simulink model "mecanique"  (Simulink 6.0)
settings: Solver=ode45  StartTime=0.0  StopTime=10.0  RelTol=1e-3
libraries: mblibv1 x11, simulink x4
settings Model: LastModifiedBy=sebastien

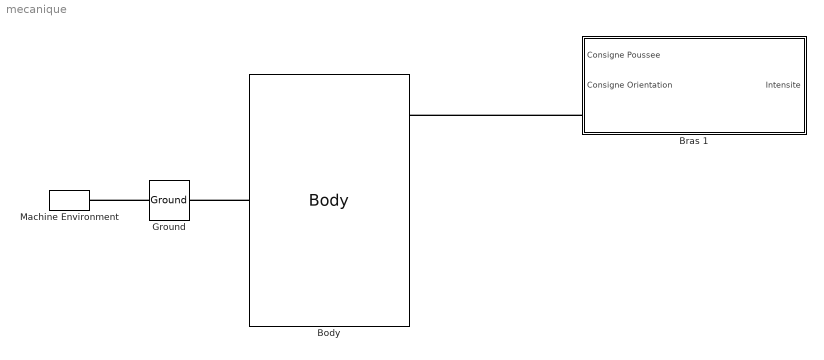
== system mecanique ==
  Body : mblibv1/Bodies/Body  PhysicalDomain=mechanical  SubClassName=Unknown  LeftPortType=workingframe  RightPortType=workingframe  LConnTagsString=CS1  RConnTagsString=CS2|CS3|CS4  DialogClass=MechanicalBodyBlock  Mass=1  MassUnits=kg  InertiaUnits=kg*m^2  Inertia=eye(3)  Shape=Cylinder  ShapeDims=[1 1]  ShapeUnits=m  ShapeUse=false  Density=1  DensityUnits=kg/m^3  DensityUse=false  CG=Left$CG$[0 0 0]$WORLD$WORLD$m$[0 0 0]$Euler X-Y-Z$deg$WORLD$false  WorkingFrames=Left$CS1$[0 0 0]$CG$CG$m$[0 0 0]$Euler X-Y-Z$deg$WORLD$true#Right$CS2$[0 0 0]$CG$CG$m$[0 0 0]$Euler X-Y-Z$deg$WORLD$true#Right$CS3$[0 0 0]$CG$CG$m$[0 0 120]$Euler X-Y-Z$deg$WORLD$true#Right$CS4$[0 0 0]$CG$CG$m$[0 0 240]$Euler X-Y-Z$deg$WORLD$true
  Bras 1 : Subsystem
  Ground : mblibv1/Bodies/Ground  Opaque=on  LeftPortType=env  RightPortType=workingframe  PhysicalDomain=Mechanical  DialogClass=GroundBlock  CoordPosition=[0 0 0]  CoordPositionUnits=m  StateVectorMgrId=-1  MachineId=[0 0]  ShowEnvPort=on
  Machine Environment : mblibv1/Bodies/Machine Environment  Tag=Factory ground  DialogController=MECH.DialogSource  Opaque=on  PortType=env  PhysicalDomain=Mechanical  DialogTemplateClass=MECH.MachineEnvironment  SyncWhenCopied=off  Gravity=[0 0 -9.81]  GravityUnits=m/s^2  GravityAsSignal=off  Dimensionality=Auto-detect  AnalysisType=Forward dynamics  LinearAssemblyTolerance=1e-3  LinearAssemblyToleranceUnits=m  AngularAssemblyTolerance=1e-3  AngularAssemblyToleranceUnits=rad  ConstraintSolverType=Stabilizing  ConstraintRelTolerance=1e-4  ConstraintAbsTolerance=1e-4  UseRobustSingularityHandling=off  StatePerturbationType=Fixed  PerturbationSize=1e-5  VisualizeMachine=on
  connections:
  Ground/LConn1 -- Machine Environment/RConn1
  Bras 1/LConn1 -- Body/RConn1
  Body/LConn1 -- Ground/RConn1

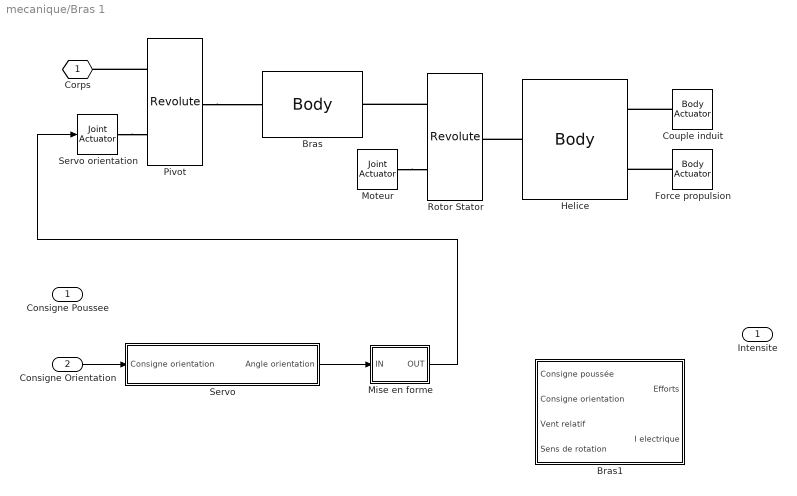
== system mecanique/Bras 1 ==
  Consigne Poussee : Inport  Port=1  LatchInput=off
  Consigne Orientation : Inport  Port=2  LatchInput=off
  Bras : mblibv1/Bodies/Body  PhysicalDomain=mechanical  SubClassName=Unknown  LeftPortType=workingframe  RightPortType=workingframe  LConnTagsString=CS1  RConnTagsString=CS2  DialogClass=MechanicalBodyBlock  Mass=1  MassUnits=kg  InertiaUnits=kg*m^2  Inertia=eye(3)  Shape=Cylinder  ShapeDims=[1 1]  ShapeUnits=m  ShapeUse=false  Density=1  DensityUnits=kg/m^3  DensityUse=false  CG=Left$CG$[0 0 0]$WORLD$WORLD$m$[0 0 0]$Euler X-Y-Z$deg$WORLD$false  WorkingFrames=Left$CS1$[0 0 0]$CG$CG$m$[0 0 0]$Euler X-Y-Z$deg$WORLD$true#Right$CS2$[0 0 0]$CG$CG$m$[0 0 0]$Euler X-Y-Z$deg$WORLD$true
  Bras1 : Subsystem
  Couple induit : mblibv1/Sensors &  Actuators/Body Actuator  Orientation=left  Opaque=on  PhysicalDomain=Mechanical  PortType=blob  ActuationStyle=Force  AngleUnits=deg  ArcVelocityUnits=deg/s  ArcAccelerationUnits=deg/s^2  CoordPositionUnits=m  VelocityUnits=m/s  AccelerationUnits=m/s^2  ForceUnits=N  TorqueUnits=N-m  ActiveIO=off  Width=1  DialogClass=MechanicalActuatorBlock  ReferenceFrame=Local (Body CS)  Angle=off  CoordPosition=on  Force=off  Torque=on
  Force propulsion : mblibv1/Sensors &  Actuators/Body Actuator  Orientation=left  Opaque=on  PhysicalDomain=Mechanical  PortType=blob  ActuationStyle=Force  AngleUnits=deg  ArcVelocityUnits=deg/s  ArcAccelerationUnits=deg/s^2  CoordPositionUnits=m  VelocityUnits=m/s  AccelerationUnits=m/s^2  ForceUnits=N  TorqueUnits=N-m  ActiveIO=off  Width=1  DialogClass=MechanicalActuatorBlock  ReferenceFrame=Local (Body CS)  Angle=off  CoordPosition=on  Force=on  Torque=off
  Helice : mblibv1/Bodies/Body  PhysicalDomain=mechanical  SubClassName=Unknown  LeftPortType=workingframe  RightPortType=workingframe  LConnTagsString=CS1  RConnTagsString=CS2|CS3  DialogClass=MechanicalBodyBlock  Mass=1  MassUnits=kg  InertiaUnits=kg*m^2  Inertia=eye(3)  Shape=Cylinder  ShapeDims=[1 1]  ShapeUnits=m  ShapeUse=false  Density=1  DensityUnits=kg/m^3  DensityUse=false  CG=Left$CG$[0 0 0]$WORLD$WORLD$m$[0 0 0]$Euler X-Y-Z$deg$WORLD$false  WorkingFrames=Left$CS1$[0 0 0]$CG$CG$m$[0 0 0]$Euler X-Y-Z$deg$WORLD$true#Right$CS2$[0 0 0]$CG$CG$m$[0 0 0]$Euler X-Y-Z$deg$WORLD$true#Right$CS3$[0 0 0]$CG$CG$m$[0 0 0]$Euler X-Y-Z$deg$WORLD$true
  Mise en forme : Subsystem
  Moteur : mblibv1/Sensors &  Actuators/Joint Actuator  Opaque=on  PhysicalDomain=Mechanical  PortType=blob  ActuationStyle=Motion  AngleUnits=rad  ArcVelocityUnits=rad/s  ArcAccelerationUnits=rad/s^2  CoordPositionUnits=m  VelocityUnits=m/s  AccelerationUnits=m/s^2  ForceUnits=N  TorqueUnits=N-m  ActiveIO=off  Width=1  DialogClass=MechanicalActuatorBlock  Primitive=R1  ReferenceFrame=Absolute (INERTIAL)
  Pivot : mblibv1/Joints/Revolute  PhysicalDomain=mechanical  SubClassName=Unknown  LeftPortType=blob  RightPortType=blob  LConnTagsString=__newl0|SA1  RConnTagsString=__newr0  NumSAPorts=1  CutJoint=off  MarkAsCut=off  Primitives=revolute  PrimitiveProps=R1$Base$[1 0 0]$revolute  DialogClass=JointBlock
  Rotor Stator : mblibv1/Joints/Revolute  PhysicalDomain=mechanical  SubClassName=Unknown  LeftPortType=blob  RightPortType=blob  LConnTagsString=__newl0|SA1  RConnTagsString=__newr0  NumSAPorts=1  CutJoint=off  MarkAsCut=off  Primitives=revolute  PrimitiveProps=R1$Base$[1 0 0]$revolute  DialogClass=JointBlock
  Servo : Subsystem
  Servo orientation : mblibv1/Sensors &  Actuators/Joint Actuator  Opaque=on  PhysicalDomain=Mechanical  PortType=blob  ActuationStyle=Motion  AngleUnits=rad  ArcVelocityUnits=rad/s  ArcAccelerationUnits=rad/s^2  CoordPositionUnits=m  VelocityUnits=m/s  AccelerationUnits=m/s^2  ForceUnits=N  TorqueUnits=N-m  ActiveIO=off  Width=1  DialogClass=MechanicalActuatorBlock  Primitive=R1  ReferenceFrame=Absolute (INERTIAL)
  Corps : PMIOPort  Tag=PMCPort  Port=1  Side=Left
  Intensite : Outport
  wires:
  Consigne Orientation/1 -> Servo/1(Consigne orientation)
  Servo/1(Angle orientation) -> Mise en forme/1(IN)
  Mise en forme/1(OUT) -> Servo orientation/1
  connections:
  Pivot/LConn1 -- Corps/RConn1
  Pivot/RConn1 -- Bras/LConn1
  Rotor Stator/LConn1 -- Bras/RConn1
  Helice/LConn1 -- Rotor Stator/RConn1
  Servo orientation/RConn1 -- Pivot/LConn2
  Couple induit/RConn1 -- Helice/RConn1
  Force propulsion/RConn1 -- Helice/RConn2
  Moteur/RConn1 -- Rotor Stator/LConn2

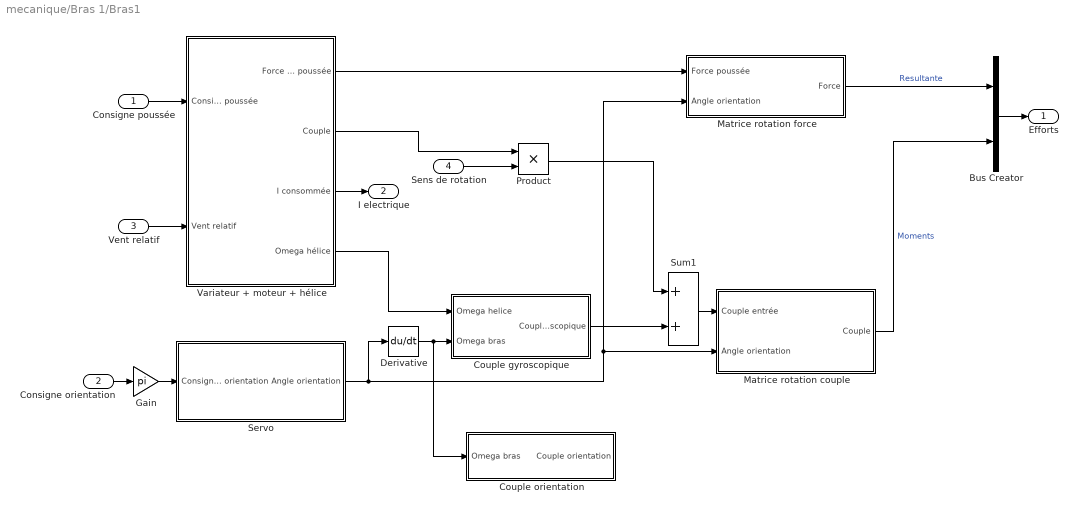
== system mecanique/Bras 1/Bras1 ==
  Consigne poussée : Inport  Port=1  LatchInput=off
  Consigne orientation : Inport  Port=2  LatchInput=off
  Vent relatif : Inport  Port=3  LatchInput=off
  Sens de rotation : Inport  Port=4  LatchInput=off
  " Couple orientation" : Subsystem
  Bus Creator : BusCreator  DialogController=Simulink.DDGSource_Bus  Inputs=2
  Couple gyroscopique : Subsystem
  Derivative : Derivative
  Gain : Gain  Gain=pi
  Matrice rotation couple : Subsystem
  Matrice rotation force : Subsystem
  Product : Product  RndMeth=Zero
  Servo : Subsystem
  Sum1 : Sum
  Variateur + moteur + hélice : Subsystem
  Efforts : Outport
  I electrique : Outport  Port=2
  wires:
  Consigne poussée/1 -> Variateur + moteur + hélice/1(Consigne poussée)
  Servo/1(Angle orientation) -> Derivative/1, Matrice rotation force/2(Angle orientation), Matrice rotation couple/2(Angle orientation)
  Matrice rotation force/1(Force) -> Bus Creator/1  "Resultante"
  Matrice rotation couple/1(Couple) -> Bus Creator/2  "Moments"
  Derivative/1 -> Couple gyroscopique/2(Omega bras), " Couple orientation"/1(Omega bras)
  Sum1/1 -> Matrice rotation couple/1(Couple entrée)
  Couple gyroscopique/1(Couple gyroscopique) -> Sum1/2
  Bus Creator/1 -> Efforts/1
  Consigne orientation/1 -> Gain/1
  Vent relatif/1 -> Variateur + moteur + hélice/2(Vent relatif)
  Variateur + moteur + hélice/1(Force de poussée) -> Matrice rotation force/1(Force poussée)
  Variateur + moteur + hélice/3(I consommée) -> I electrique/1
  Variateur + moteur + hélice/4(Omega hélice) -> Couple gyroscopique/1(Omega helice)
  Gain/1 -> Servo/1(Consigne orientation)
  Sens de rotation/1 -> Product/2
  Product/1 -> Sum1/1
  Variateur + moteur + hélice/2(Couple) -> Product/1

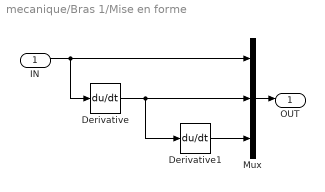
== system mecanique/Bras 1/Mise en forme ==
  IN : Inport  Port=1  LatchInput=off
  Derivative : Derivative
  Derivative1 : Derivative
  Mux : Mux  Inputs=3
  OUT : Outport
  wires:
  Derivative/1 -> Mux/2, Derivative1/1
  IN/1 -> Derivative/1, Mux/1
  Derivative1/1 -> Mux/3
  Mux/1 -> OUT/1

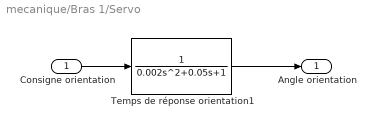
== system mecanique/Bras 1/Servo ==
  Consigne orientation : Inport  Port=1  LatchInput=off
  Temps de réponse orientation1 : TransferFcn  Denominator=[ 0.002 0.05 1]
  Angle orientation : Outport
  wires:
  Consigne orientation/1 -> Temps de réponse orientation1/1
  Temps de réponse orientation1/1 -> Angle orientation/1

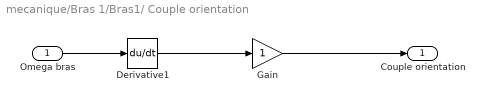
== system mecanique/Bras 1/Bras1/ Couple orientation ==
  Omega bras : Inport  Port=1  LatchInput=off
  Derivative1 : Derivative
  Gain : Gain
  Couple orientation : Outport
  wires:
  Omega bras/1 -> Derivative1/1
  Derivative1/1 -> Gain/1
  Gain/1 -> Couple orientation/1

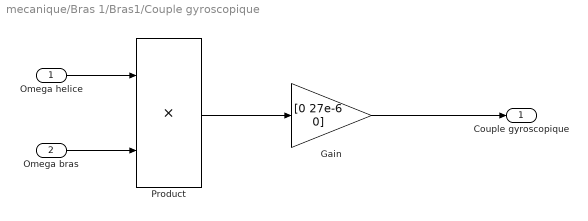
== system mecanique/Bras 1/Bras1/Couple gyroscopique ==
  Omega helice : Inport  Port=1  LatchInput=off
  Omega bras : Inport  Port=2  LatchInput=off
  Gain : Gain  Gain=[0 27e-6 0]
  Product : Product  RndMeth=Zero
  Couple gyroscopique : Outport
  wires:
  Omega helice/1 -> Product/1
  Omega bras/1 -> Product/2
  Product/1 -> Gain/1
  Gain/1 -> Couple gyroscopique/1

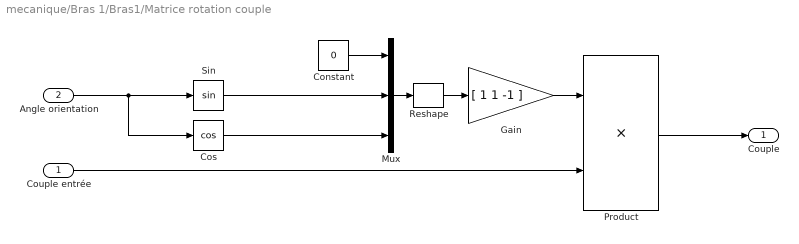
== system mecanique/Bras 1/Bras1/Matrice rotation couple ==
  Couple entrée : Inport  Port=1  LatchInput=off
  Angle orientation : Inport  Port=2  LatchInput=off
  Constant : Constant  Value=0
  Cos : Trigonometry  Operator=cos
  Gain : Gain  Gain=[ 1 1 -1 ]
  Mux : Mux  Inputs=3
  Product : Product  RndMeth=Zero
  Reshape : simulink/Math Operations/Reshape  OutputDimensionality=1-D array  OutputDimensions=[1,1]
  Sin : Trigonometry
  Couple : Outport
  wires:
  Angle orientation/1 -> Cos/1, Sin/1
  Constant/1 -> Mux/1
  Cos/1 -> Mux/3
  Sin/1 -> Mux/2
  Mux/1 -> Reshape/1
  Gain/1 -> Product/1
  Couple entrée/1 -> Product/2
  Product/1 -> Couple/1
  Reshape/1 -> Gain/1

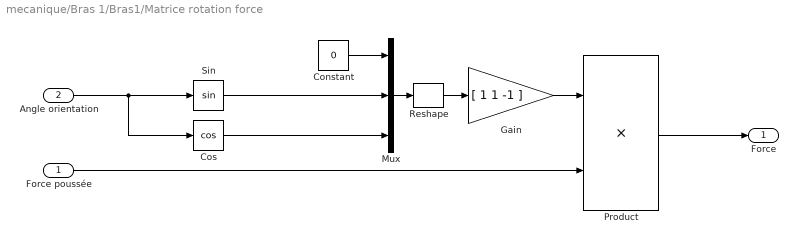
== system mecanique/Bras 1/Bras1/Matrice rotation force ==
  Force poussée : Inport  Port=1  LatchInput=off
  Angle orientation : Inport  Port=2  LatchInput=off
  Constant : Constant  Value=0
  Cos : Trigonometry  Operator=cos
  Gain : Gain  Gain=[ 1 1 -1 ]
  Mux : Mux  Inputs=3
  Product : Product  RndMeth=Zero
  Reshape : simulink/Math Operations/Reshape  OutputDimensionality=1-D array  OutputDimensions=[1,1]
  Sin : Trigonometry
  Force : Outport
  wires:
  Angle orientation/1 -> Cos/1, Sin/1
  Constant/1 -> Mux/1
  Cos/1 -> Mux/3
  Sin/1 -> Mux/2
  Mux/1 -> Reshape/1
  Gain/1 -> Product/1
  Force poussée/1 -> Product/2
  Product/1 -> Force/1
  Reshape/1 -> Gain/1

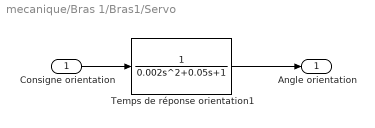
== system mecanique/Bras 1/Bras1/Servo ==
  Consigne orientation : Inport  Port=1  LatchInput=off
  Temps de réponse orientation1 : TransferFcn  Denominator=[ 0.002 0.05 1]
  Angle orientation : Outport
  wires:
  Consigne orientation/1 -> Temps de réponse orientation1/1
  Temps de réponse orientation1/1 -> Angle orientation/1

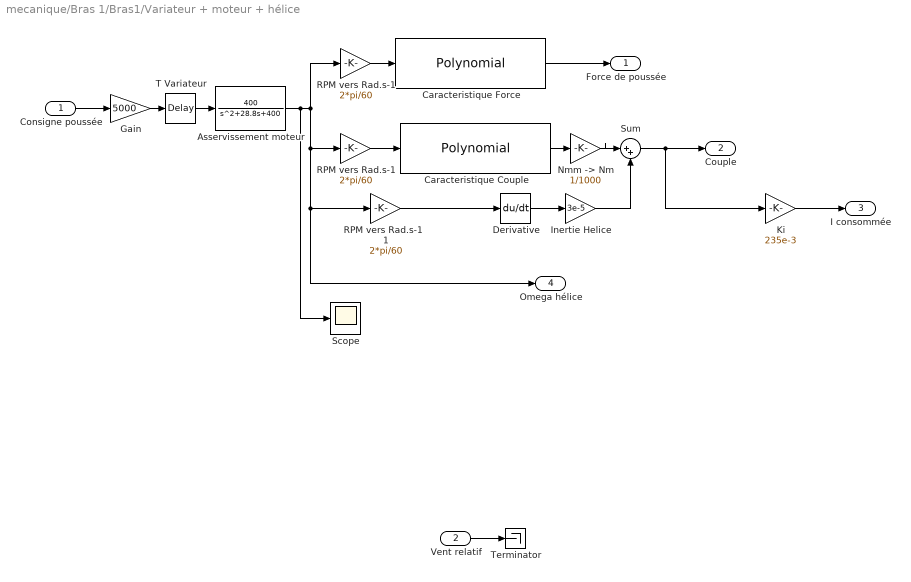
== system mecanique/Bras 1/Bras1/Variateur + moteur + hélice ==
  Consigne poussée : Inport  Port=1  LatchInput=off
  Vent relatif : Inport  Port=2  LatchInput=off
  Asservissement moteur : TransferFcn  Numerator=[400]  Denominator=[1 28.8 400]
  Caracteristique Couple : simulink/Math Operations/Polynomial  coefs="[3.323e-4  -3.102e-2 1.84e-1]"
  Caracteristique Force : simulink/Math Operations/Polynomial  coefs=[2e-5 -1e-3 2e-3]
  Derivative : Derivative
  Gain : Gain  Gain=5000
  Inertie Helice : Gain  Gain=3e-5
  Ki : Gain  Gain=235e-3
  "Nmm -> Nm" : Gain  Gain=1/1000
  RPM vers Rad.s-1 : Gain  Gain=2*pi/60
  "RPM vers Rad.s-1   " : Gain  Gain=2*pi/60
  RPM vers Rad.s-1   1 : Gain  Gain=2*pi/60
  Scope : Scope
      settings: YMin=4990  YMax=5130  SaveName=ScopeData6
  Sum : Sum  Inputs=|++
  T Variateur : TransportDelay  DelayTime=20e-3
  Terminator : Terminator
  Force de poussée : Outport
  Couple : Outport  Port=2
  I consommée : Outport  Port=3
  Omega hélice : Outport  Port=4
  wires:
  Vent relatif/1 -> Terminator/1
  Consigne poussée/1 -> Gain/1
  Caracteristique Force/1 -> Force de poussée/1
  T Variateur/1 -> Asservissement moteur/1
  Asservissement moteur/1 -> Omega hélice/1, RPM vers Rad.s-1   1/1, "RPM vers Rad.s-1   "/1, RPM vers Rad.s-1/1, Scope/1
  Derivative/1 -> Inertie Helice/1
  Caracteristique Couple/1 -> "Nmm -> Nm"/1
  Sum/1 -> Ki/1, Couple/1
  Inertie Helice/1 -> Sum/2
  Ki/1 -> I consommée/1
  Gain/1 -> T Variateur/1
  RPM vers Rad.s-1/1 -> Caracteristique Force/1
  "RPM vers Rad.s-1   "/1 -> Caracteristique Couple/1
  "Nmm -> Nm"/1 -> Sum/1
  RPM vers Rad.s-1   1/1 -> Derivative/1
